simulink model "soft_switch_turbine_sim"  (R2025b)
settings: Solver=ode23s  StartTime=0.0  StopTime=T_sim  MaxStep=1e-6  RelTol=1e-5
InitFcn:
  | run param_file_turbine.m
values from neighbouring files (symbols this model uses):
  param = struct()    [Copy_of_param_file.m]    (also in param_file.m; param_file_loss_vs_freq.m; param_file_original.m; param_file_turbine.m)
settings Model: Creator=user  LastModifiedBy=user
settings SolverCC: ZeroCrossAlgorithm=Adaptive
settings DebuggingCC: IgnoredZcDiagnostic=none

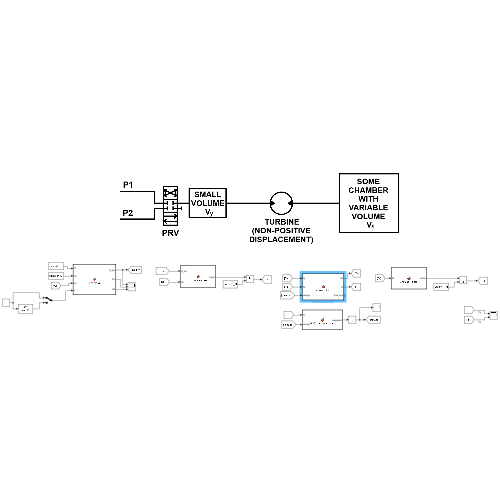
[thumbnail: Simulink's stored preview of the top-level diagram]
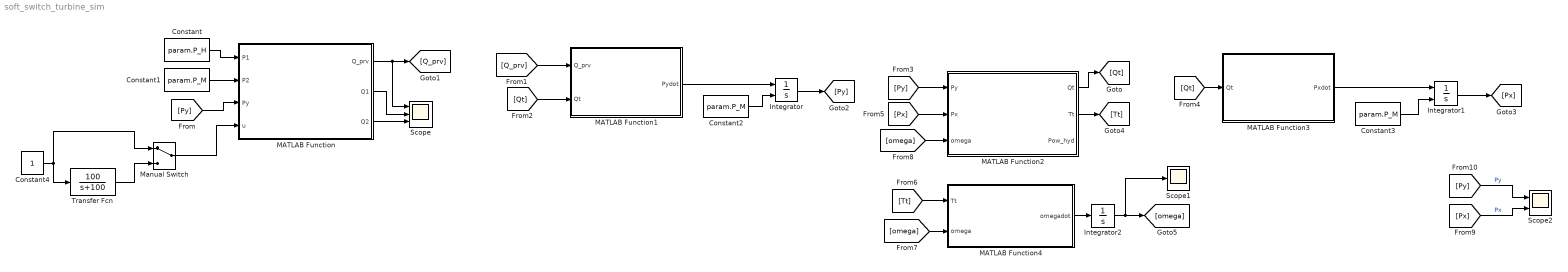
== system soft_switch_turbine_sim ==
  Constant : Constant  Value=param.P_H
  Constant1 : Constant  Value=param.P_M
  Constant2 : Constant  Value=param.P_M
  Constant3 : Constant  Value=param.P_M
  Constant4 : Constant
  Integrator : Integrator  InitialConditionSource=external
  Integrator1 : Integrator  InitialConditionSource=external
  Integrator2 : Integrator
  MATLAB Function : MATLAB Function  TreatAsAtomicUnit=on
  MATLAB Function1 : MATLAB Function  TreatAsAtomicUnit=on
  MATLAB Function2 : MATLAB Function  TreatAsAtomicUnit=on
  MATLAB Function3 : MATLAB Function  TreatAsAtomicUnit=on
  MATLAB Function4 : MATLAB Function  TreatAsAtomicUnit=on
  Manual Switch : ManualSwitch
  Scope : Scope  NumInputPorts=3
  Scope1 : Scope
      settings: ActiveDisplayYMinimum=-1  ActiveDisplayYMaximum=1
  Scope2 : Scope  NumInputPorts=2
      settings: ActiveDisplayYMinimum=2.5851192689889371E+6  ActiveDisplayYMaximum=1.1203926579099566E+7  DataLoggingVariableName=ScopeData2
  Transfer Fcn : TransferFcn  Numerator=[100]  Denominator=[1 100]
  wires:
  Constant/1 -> MATLAB Function/1(P1)
  Constant1/1 -> MATLAB Function/2(P2)
  [Py] -> MATLAB Function/3(Py)
  MATLAB Function/3(Q2) -> Scope/3
  MATLAB Function/2(Q1) -> Scope/2
  MATLAB Function/1(Q_prv) -> [Q_prv], Scope/1
  MATLAB Function1/1(Pydot) -> Integrator/1
  Constant2/1 -> Integrator/2
  MATLAB Function2/1(Qt) -> [Qt]
  [Q_prv] -> MATLAB Function1/1(Q_prv)
  [Qt] -> MATLAB Function1/2(Qt)
  Integrator/1 -> [Py]
  [Py] -> MATLAB Function2/1(Py)
  [Qt] -> MATLAB Function3/1(Qt)
  MATLAB Function3/1(Pxdot) -> Integrator1/1
  Constant3/1 -> Integrator1/2
  Integrator1/1 -> [Px]
  [Px] -> MATLAB Function2/2(Px)
  MATLAB Function2/2(Tt) -> [Tt]
  [Tt] -> MATLAB Function4/1(Tt)
  MATLAB Function4/1(omegadot) -> Integrator2/1
  Integrator2/1 -> [omega], Scope1/1
  [omega] -> MATLAB Function4/2(omega)
  [omega] -> MATLAB Function2/3(omega)
  Constant4/1 -> Manual Switch/1, Transfer Fcn/1
  Transfer Fcn/1 -> Manual Switch/2
  Manual Switch/1 -> MATLAB Function/4(u)
  [Px] -> Scope2/2  "Px"
  [Py] -> Scope2/1  "Py"

== matlab function soft_switch_turbine_sim/MATLAB Function1 ==
  data: Q_prv input; Pydot output; Qt input; param parameter
function Pydot = small_volume_block(Q_prv, Qt, param)

% Pressure dynamics of small intermediate volume Vy
Pydot = param.beta/param.Vy_0*(Q_prv - Qt);

end

== matlab function soft_switch_turbine_sim/MATLAB Function ==
  data: P1 input; P2 input; Py input; u input; Q_prv output; Q1 output; Q2 output; param parameter
function [Q_prv, Q1, Q2] = prv_block(P1, P2, Py, u, param)

% Limit command
u = max(-1, min(1, u));

% Split command
u1 = max(u, 0);      % P1 side opening
u2 = max(-u, 0);     % P2 side opening

% Valve areas
Av1 = param.max_Av*u1;
Av2 = param.max_Av*u2;

% Pressure drops from rails to small volume
dP1 = P1 - Py;
dP2 = P2 - Py;

% Flows into small volume
Q1 = param.Cd*Av1*sqrt(2*abs(dP1)/param.rho)*sign(dP1);
Q2 = param.Cd*Av2*sqrt(2*abs(dP2)/param.rho)*sign(dP2);

% Total flow into Vy
Q_prv = Q1 + Q2;

end

== matlab function soft_switch_turbine_sim/MATLAB Function2 ==
  data: Py input; Qt output; Px input; omega input; Tt output; Pow_hyd output; param parameter
function [Qt, Tt, Pow_hyd] = turbine_block(Py, Px, omega, param)

% Pressure drop across turbine
dP_t = Py - Px;

% Flow through turbine
Qt = param.Cd*param.At*sqrt(2*abs(dP_t)/param.rho)*sign(dP_t);

% Hydraulic power
Pow_hyd = dP_t*Qt;

% Simple turbine torque model
Tt = param.K_turbine*Pow_hyd;

% Optional speed damping inside turbine
Tt = Tt - param.B_turbine*omega;

end

== matlab function soft_switch_turbine_sim/MATLAB Function3 ==
  data: Qt input; Pxdot output; param parameter
function Pxdot = chamber_block(Qt, param)

% Pressure dynamics of variable chamber Vx
Pxdot = (param.beta/param.Vx_0)*(Qt);

end

== matlab function soft_switch_turbine_sim/MATLAB Function4 ==
  data: Tt input; omegadot output; omega input; param parameter
function omegadot = shaft_dynamics_block(Tt, omega, param)

% Shaft dynamics with no external torque
omegadot = (Tt - param.B_shaft*omega)/param.J_total;

end
